simulink model "TransmissionController"  (R2023a)
settings: configuration reference "VehicleFixed10ms" (kept outside this file)
StartFcn:
  | %tic
StopFcn:
  | %toc
libraries: autolibtranscontrolscommon x1
settings Model: DataDictionary=VirtualVehicleTemplate.sldd  ModifiedByFormat=The MathWorks, Inc.  Creator=The MathWorks, Inc.  LastModifiedBy=The MathWorks, Inc.
settings ConfigSetRef: SourceName=VehicleFixed10ms

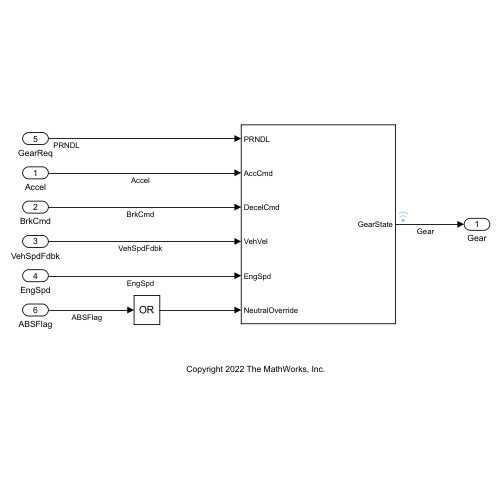
[thumbnail: Simulink's stored preview of the top-level diagram]
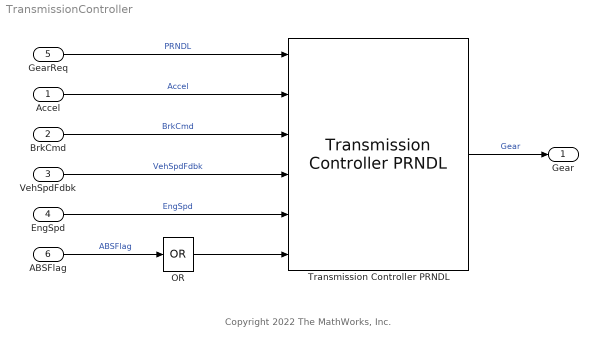
== system TransmissionController ==
  note: Copyright 2022 The MathWorks, Inc.
  Accel : Inport  OutDataTypeStr=double  PortDimensions=1
  BrkCmd : Inport  Port=2  OutDataTypeStr=double  PortDimensions=1
  VehSpdFdbk : Inport  Port=3  OutDataTypeStr=double  Unit=m/s  PortDimensions=1
  EngSpd : Inport  Port=4  OutDataTypeStr=double  Unit=rad/s  PortDimensions=1
  GearReq : Inport  Port=5  OutDataTypeStr=double  PortDimensions=1
  ABSFlag : Inport  Port=6  OutDataTypeStr=boolean  PortDimensions=4
  OR : Logic  Operator=OR  Inputs=1  AllPortsSameDT=off  OutDataTypeStr=boolean
  Transmission Controller PRNDL : autolibtranscontrolscommon/Transmission Controller PRNDL  DriveMode=off  GearInit=CtrlTcuInitGear  LugSpd=CtrlTcuLugSpd  MinUpSpd=CtrlTcuMinUpSpd  tClutchUp=CtrlTcuTmUpSh  tClutchDn=CtrlTcuTmDnSh  tPark=120  VelUnit=km/hr  UpShSpd=CtrlTcuUpShSpd  UpLdBpt=CtrlTcuUpLdBpt  UpShBpt=1:7  UpPtBpt=[1 2]  DnShfSpd=CtrlTcuDnShSpd  DnShSpd=CtrlTcuDnShSpd  DnLdBpt=CtrlTcuDnLdBpt  DnShBpt=2:8  DnPtBpt=[1 2]  POFS=zeros(4,1)  GOFS=zeros(1,7)  Ngears=8  aMode=6
  Gear : Outport  OutDataTypeStr=double  PortDimensions=1  VectorParamsAs1DForOutWhenUnconnected=off
  wires:
  ABSFlag/1 -> OR/1  "ABSFlag"
  Transmission Controller PRNDL/1 -> Gear/1  "Gear"
  GearReq/1 -> Transmission Controller PRNDL/1  "PRNDL"
  Accel/1 -> Transmission Controller PRNDL/2  "Accel"
  BrkCmd/1 -> Transmission Controller PRNDL/3  "BrkCmd"
  EngSpd/1 -> Transmission Controller PRNDL/5  "EngSpd"
  VehSpdFdbk/1 -> Transmission Controller PRNDL/4  "VehSpdFdbk"
  OR/1 -> Transmission Controller PRNDL/6
